simulink library "INT_InjSys_CtlQnt"  (R2016b)
settings: Solver=VariableStepAuto  StartTime=0.0  StopTime=10.0  RelTol=1e-3
settings Model: Creator=mayongchao  LastModifiedBy=mayongchao

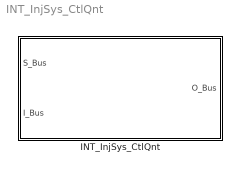
== system INT_InjSys_CtlQnt ==
  INT_InjSys_CtlQnt : Subsystem

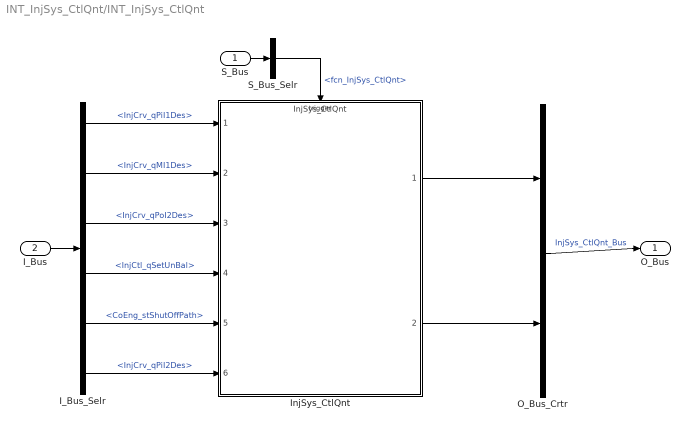
== system INT_InjSys_CtlQnt/INT_InjSys_CtlQnt ==
  S_Bus : Inport
  I_Bus : Inport  Port=2
  I_Bus_Selr : BusSelector  OutputSignals=InjCrv_qPiI1Des,InjCrv_qMI1Des,InjCrv_qPoI2Des,InjCtl_qSetUnBal,CoEng_stShutOffPath,InjCrv_qPiI2Des
  InjSys_CtlQnt : ModelReference  ModelNameDialog=InjSys_CtlQnt  SimulationMode=Normal  ModelReferenceVersion=1.5  TriggerPortName=function  TriggerPortTriggerType=function-call  TriggerPortStatesWhenEnabling=held
  O_Bus_Crtr : BusCreator  Inputs=2
  S_Bus_Selr : BusSelector  OutputSignals=fcn_InjSys_CtlQnt
  O_Bus : Outport
  wires:
  S_Bus_Selr/1 -> InjSys_CtlQnt/Trigger  "<fcn_InjSys_CtlQnt>"
  S_Bus/1 -> S_Bus_Selr/1
  I_Bus/1 -> I_Bus_Selr/1
  I_Bus_Selr/1 -> InjSys_CtlQnt/1  "<InjCrv_qPiI1Des>"
  I_Bus_Selr/2 -> InjSys_CtlQnt/2  "<InjCrv_qMI1Des>"
  I_Bus_Selr/3 -> InjSys_CtlQnt/3  "<InjCrv_qPoI2Des>"
  I_Bus_Selr/4 -> InjSys_CtlQnt/4  "<InjCtl_qSetUnBal>"
  I_Bus_Selr/5 -> InjSys_CtlQnt/5  "<CoEng_stShutOffPath>"
  I_Bus_Selr/6 -> InjSys_CtlQnt/6  "<InjCrv_qPiI2Des>"
  O_Bus_Crtr/1 -> O_Bus/1  "InjSys_CtlQnt_Bus"
  InjSys_CtlQnt/1 -> O_Bus_Crtr/1
  InjSys_CtlQnt/2 -> O_Bus_Crtr/2
